simulink model "Veh"  (R2018a)
settings: configuration reference "cs_ert" (kept outside this file)
settings Model: DataDictionary=Veh.sldd  Creator=zhoutinglin  LastModifiedBy=zhoutinglin

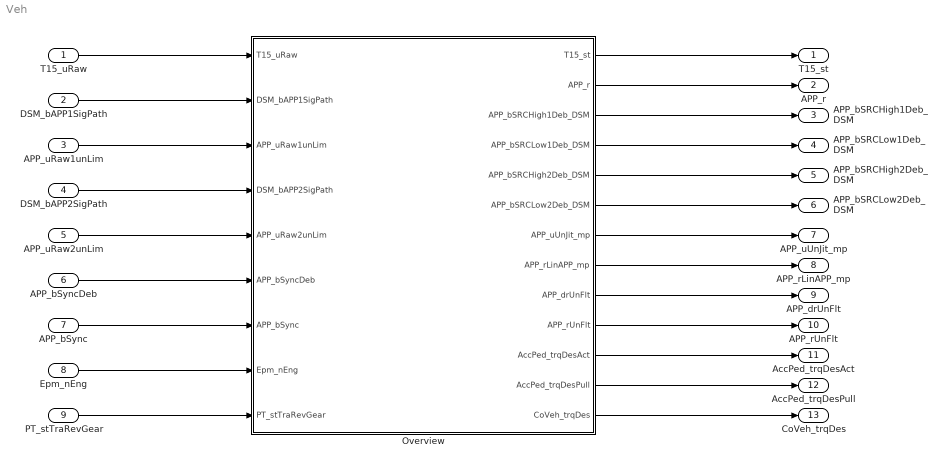
== system Veh ==
  T15_uRaw : Inport
  DSM_bAPP1SigPath : Inport  Port=2
  APP_uRaw1unLim : Inport  Port=3
  DSM_bAPP2SigPath : Inport  Port=4
  APP_uRaw2unLim : Inport  Port=5
  APP_bSyncDeb : Inport  Port=6
  APP_bSync : Inport  Port=7
  Epm_nEng : Inport  Port=8
  PT_stTraRevGear : Inport  Port=9
  Overview : Subsystem
  T15_st : Outport
  APP_r : Outport  Port=2
  APP_bSRCHigh1Deb_DSM : Outport  Port=3
  APP_bSRCLow1Deb_DSM : Outport  Port=4
  APP_bSRCHigh2Deb_DSM : Outport  Port=5
  APP_bSRCLow2Deb_DSM : Outport  Port=6
  APP_uUnJit_mp : Outport  Port=7
  APP_rLinAPP_mp : Outport  Port=8
  APP_drUnFlt : Outport  Port=9
  APP_rUnFlt : Outport  Port=10
  AccPed_trqDesAct : Outport  Port=11
  AccPed_trqDesPull : Outport  Port=12
  CoVeh_trqDes : Outport  Port=13
  wires:
  T15_uRaw/1 -> Overview/1(T15_uRaw)
  DSM_bAPP1SigPath/1 -> Overview/2(DSM_bAPP1SigPath)
  APP_uRaw1unLim/1 -> Overview/3(APP_uRaw1unLim)
  DSM_bAPP2SigPath/1 -> Overview/4(DSM_bAPP2SigPath)
  APP_uRaw2unLim/1 -> Overview/5(APP_uRaw2unLim)
  APP_bSyncDeb/1 -> Overview/6(APP_bSyncDeb)
  APP_bSync/1 -> Overview/7(APP_bSync)
  Epm_nEng/1 -> Overview/8(Epm_nEng)
  PT_stTraRevGear/1 -> Overview/9(PT_stTraRevGear)
  Overview/1(T15_st) -> T15_st/1
  Overview/2(APP_r) -> APP_r/1
  Overview/3(APP_bSRCHigh1Deb_DSM) -> APP_bSRCHigh1Deb_DSM/1
  Overview/4(APP_bSRCLow1Deb_DSM) -> APP_bSRCLow1Deb_DSM/1
  Overview/5(APP_bSRCHigh2Deb_DSM) -> APP_bSRCHigh2Deb_DSM/1
  Overview/6(APP_bSRCLow2Deb_DSM) -> APP_bSRCLow2Deb_DSM/1
  Overview/7(APP_uUnJit_mp) -> APP_uUnJit_mp/1
  Overview/8(APP_rLinAPP_mp) -> APP_rLinAPP_mp/1
  Overview/9(APP_drUnFlt) -> APP_drUnFlt/1
  Overview/10(APP_rUnFlt) -> APP_rUnFlt/1
  Overview/11(AccPed_trqDesAct) -> AccPed_trqDesAct/1
  Overview/12(AccPed_trqDesPull) -> AccPed_trqDesPull/1
  Overview/13(CoVeh_trqDes) -> CoVeh_trqDes/1

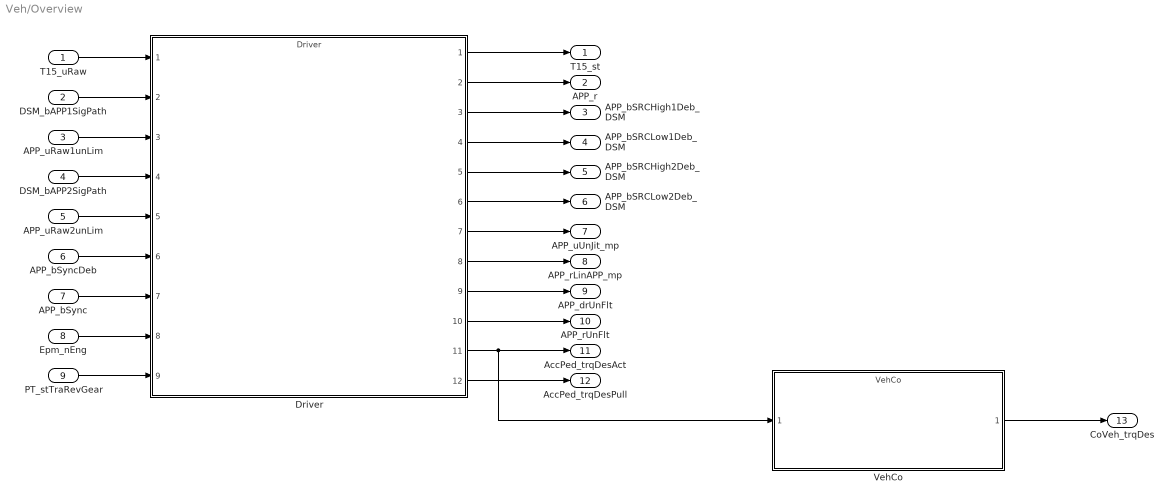
== system Veh/Overview ==
  T15_uRaw : Inport
  DSM_bAPP1SigPath : Inport  Port=2
  APP_uRaw1unLim : Inport  Port=3
  DSM_bAPP2SigPath : Inport  Port=4
  APP_uRaw2unLim : Inport  Port=5
  APP_bSyncDeb : Inport  Port=6
  APP_bSync : Inport  Port=7
  Epm_nEng : Inport  Port=8
  PT_stTraRevGear : Inport  Port=9
  Driver : ModelReference  ModelNameDialog=Driver  SimulationMode=Normal  ModelReferenceVersion=1.3
  VehCo : ModelReference  ModelNameDialog=VehCo  SimulationMode=Normal  ModelReferenceVersion=1.3
  T15_st : Outport
  APP_r : Outport  Port=2
  APP_bSRCHigh1Deb_DSM : Outport  Port=3
  APP_bSRCLow1Deb_DSM : Outport  Port=4
  APP_bSRCHigh2Deb_DSM : Outport  Port=5
  APP_bSRCLow2Deb_DSM : Outport  Port=6
  APP_uUnJit_mp : Outport  Port=7
  APP_rLinAPP_mp : Outport  Port=8
  APP_drUnFlt : Outport  Port=9
  APP_rUnFlt : Outport  Port=10
  AccPed_trqDesAct : Outport  Port=11
  AccPed_trqDesPull : Outport  Port=12
  CoVeh_trqDes : Outport  Port=13
  wires:
  Driver/11 -> VehCo/1, AccPed_trqDesAct/1
  T15_uRaw/1 -> Driver/1
  DSM_bAPP1SigPath/1 -> Driver/2
  APP_uRaw1unLim/1 -> Driver/3
  DSM_bAPP2SigPath/1 -> Driver/4
  APP_uRaw2unLim/1 -> Driver/5
  APP_bSyncDeb/1 -> Driver/6
  APP_bSync/1 -> Driver/7
  Epm_nEng/1 -> Driver/8
  PT_stTraRevGear/1 -> Driver/9
  Driver/1 -> T15_st/1
  Driver/2 -> APP_r/1
  Driver/3 -> APP_bSRCHigh1Deb_DSM/1
  Driver/4 -> APP_bSRCLow1Deb_DSM/1
  Driver/5 -> APP_bSRCHigh2Deb_DSM/1
  Driver/6 -> APP_bSRCLow2Deb_DSM/1
  Driver/7 -> APP_uUnJit_mp/1
  Driver/8 -> APP_rLinAPP_mp/1
  Driver/9 -> APP_drUnFlt/1
  Driver/10 -> APP_rUnFlt/1
  Driver/12 -> AccPed_trqDesPull/1
  VehCo/1 -> CoVeh_trqDes/1
